simulink model "Simu_Kinematics_Dynamics_Model_2014"  (R2023a)
settings: Solver=ode45  StartTime=0.0  StopTime=1000.0  RelTol=1e-3
InitFcn:
  | addpath('../parameters/')
  | simulation_parameters
  | aircraft_parameters
  | sensor_parameters
  | wind_parameters
undefined symbols (not defined in the file): drawAircraft, plotmavstatevariables
libraries: simulink x6
settings Model: Creator=h1huang  LastModifiedBy=user
settings SolverCC: AlgebraicLoopSolver=TrustRegion
settings DataIOCC: SaveFormat=StructureWithTime
settings OptimizationCC: LifeSpan=inf
settings DebuggingCC: UnconnectedInputMsg=warning  UnconnectedOutputMsg=warning  UnconnectedLineMsg=warning  SFExecutionAtInitializationDiag=none  ArithmeticOperatorsInVariantConditions=warning
settings HardwareCC: ProdBitPerSizeT=32  ProdBitPerPtrDiffT=32  ProdWordSize=32  ProdHWDeviceType=Specified
settings SFSimCC: CustomCodeUndefinedFunction=UseInterfaceOnly
settings CodeAppCC: StateflowObjectComments=on

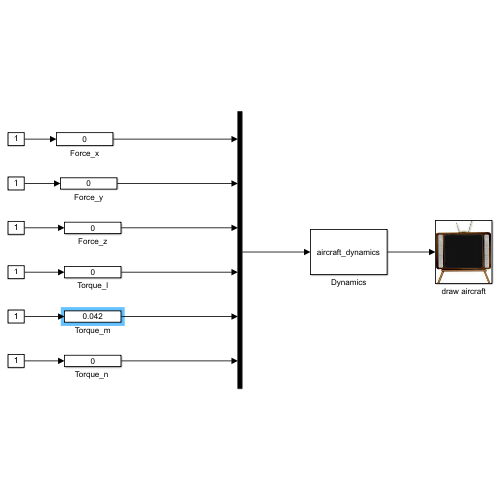
[thumbnail: Simulink's stored preview of the top-level diagram]
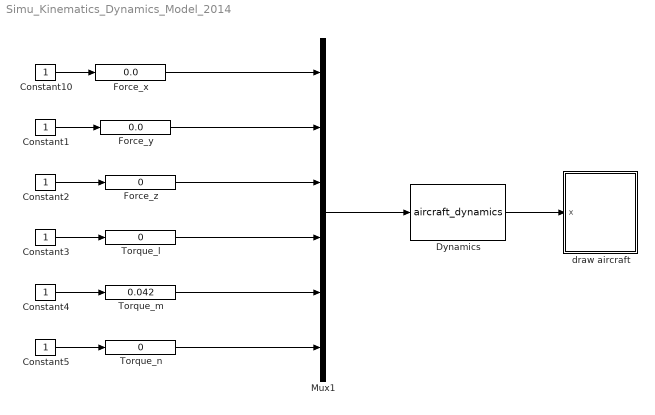
== system Simu_Kinematics_Dynamics_Model_2014 ==
  Constant{1..5,10} (6 alike) : Constant
  Dynamics : S-Function  FunctionName=aircraft_dynamics  Parameters=UAV  SFunctionDeploymentMode=off  EnableBusSupport=off
  Force_x : simulink/Math Operations/Slider Gain  gain=0.0  low=-1  high=1
  Force_y : simulink/Math Operations/Slider Gain  gain=0.0  low=-1  high=1
  Force_z : simulink/Math Operations/Slider Gain  gain=0  low=-1  high=1
  Mux1 : Mux  Inputs=6
  Torque_l : simulink/Math Operations/Slider Gain  gain=0  low=-0.1  high=0.1
  Torque_m : simulink/Math Operations/Slider Gain  gain=0.042  low=-0.1  high=0.1
  "Torque_n " : simulink/Math Operations/Slider Gain  gain=0  low=-0.1  high=0.1
  draw aircraft : Subsystem
      mask Display: image(imread('../chap2/tv.jpg'))
  wires:
  Mux1/1 -> Dynamics/1
  Constant3/1 -> Torque_l/1
  Force_x/1 -> Mux1/1
  Torque_m/1 -> Mux1/5
  Constant4/1 -> Torque_m/1
  Constant1/1 -> Force_y/1
  Force_z/1 -> Mux1/3
  Constant2/1 -> Force_z/1
  Torque_l/1 -> Mux1/4
  Force_y/1 -> Mux1/2
  "Torque_n "/1 -> Mux1/6
  Dynamics/1 -> draw aircraft/1(x)
  Constant10/1 -> Force_x/1
  Constant5/1 -> "Torque_n "/1

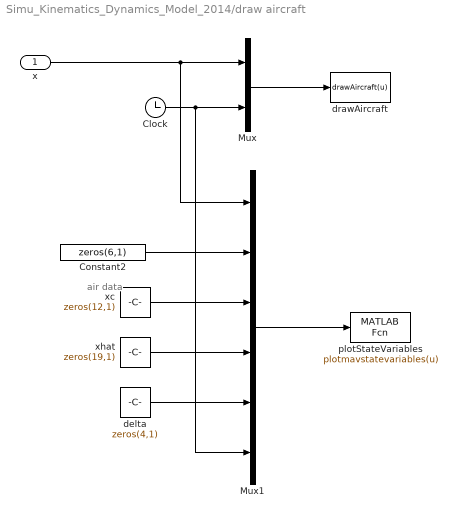
== system Simu_Kinematics_Dynamics_Model_2014/draw aircraft ==
  note: air data
  x : Inport
  Clock : Clock
  Constant2 : Constant  Value=zeros(6,1)
  Mux : Mux  Inputs=2
  Mux1 : Mux  Inputs=6
  delta : Constant  Value=zeros(4,1)
  drawAircraft : MATLABFcn  MATLABFcn=drawAircraft(u)  OutputDimensions=0  SampleTime=0.1
  plotStateVariables : MATLABFcn  MATLABFcn=plotmavstatevariables(u)  OutputDimensions=0  SampleTime=0.1
  xc : Constant  Value=zeros(12,1)
  xhat : Constant  Value=zeros(19,1)
  wires:
  Mux/1 -> drawAircraft/1
  x/1 -> Mux/1, Mux1/1
  Clock/1 -> Mux/2, Mux1/6
  Mux1/1 -> plotStateVariables/1
  xhat/1 -> Mux1/4
  xc/1 -> Mux1/3
  delta/1 -> Mux1/5
  Constant2/1 -> Mux1/2
